simulink library "DiffSteer_model"  (R2013a)
settings: Solver=ode45  StartTime=0.0  StopTime=10.0  RelTol=1e-3
settings Model: Creator=Felipe  LastModifiedBy=Felipe

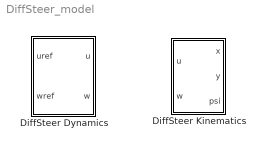
== system DiffSteer_model ==
  DiffSteer Dynamics : Subsystem  mask{umax=0.75, wmax=1.745, dumax=0.3, dwmax=1.745, param=[0.2604 0.2509 -0.000499 0.9965 0.00263 1.0768]}
      mask prompts: umax "Maximum linear velocity [m/s]"; wmax "Maximum angular velocity [rad/s]"; dumax "Maximum linear acceleration [m/s^2]"; dwmax "Maximum angular acceleration [rad/s^2]"; param "Dynamic parameters"
      mask help: Dynamics of the differential steered (unicycle-like) vehicle
      mask Help:
      | Dynamics of the differential steered (unicycle-like) vehicle.
      | 
      | This block recieves the linear and angular velocities signals (references) calculated by the robot controller and simulates the actual linear and angular velocities that the robot would have according to its dynamic parameters. It is intended to be used with the DiffSteer Kinematics block.
      | 
      | <b>Parameters:</b>
      | 
      | Maximum linear velocity (1x1): Vehicle linear velocity limit [m/s] (umax)
      | Maximum angular velocity (1x1): Vehicle angular velocity limit [rad/s] (wmax)
      | Maximum linear acceleration (1x1): Vehicle linear acceleration limit [m/s^2] (dumax)
      | Maximum angular acceleration (1x1): Vehicle angular acceleration limit [rad/s^2] (dwmax)
      | Dynamic parameters for an specific mobile robot acoording to [1-3] (1x6): (param)
      | [\theta_1 [s], \theta_2 [s], \theta_3 [sm/rad2], \theta_4, \theta_5 [s/m], \theta_6]
      | 
      | <b>Inputs::</b>
      | 
      | uref (1x1): reference for linear velocity [m/s]
      | wref (1x1): reference for angular velocity [rad/s]
      | 
      | <b>Outputs:</b>
      | 
      | u (1x1): robot linear velocity [m/s]
      | w (1x1): robot angular velocity [rad/s]
      | 
      | 
      | <b>Use:</b>
      | 
      | The inputs [uref, wref] must recieve the reference signals for linear and angular velocities.
      | 
      | The outputs [u, w] are to be conected to the inputs [u, w] of the Kinematics block.
      | 
      | 
      | <b>Notes:</b>
      | 
      | The default dynamic parameters correspond to the dynamics of the Pioneer 3-DX, from Mobile Robots, with a SICK LASER sensor mounted on its platform. To simulate the dynamics of a different robot, its parameters must be identified and input on the correspondent box.
      | 
      | The following sets of parameters were obtained via identification for some mobile robots:
      | 
      | [0.2604 0.2509 -0.000499 0.9965 0.00263 1.0768]; % Pioneer 3DX with Sick LASER sensor
      | [0.5338 0.2168 -0.0134 0.9560 -0.0843 1.0590]; % Pioneer 3DX without LASER sensor
      | [0.2183 0.1918 -0.0050 0.9993 -0.0279 1.0142]; % Pioneer 3DX (identified by Jeffrey Laut)
      | [0.1992 0.13736 0.001954 0.9907 0.01554 0.9866]; % Pioneer 2 without onboard computer (no LASER sensor)
      | [0.3037 0.2768 -0.0004018 0.9835 0.003818 1.0725]; % Pioneer 2 with onboard computer (no LASER sensor)
      | [0.3759 0.0188 0.0128 1.0027 -0.0015 0.9808]; % Robotic wheelchair carring a 55kg person
      | [0.4263 0.0289 0.0058 0.9883 0.0134 0.9931]; % Robotic wheelchair carring a 125kg person
      | [0.0228 0.0568 -0.0001 1.0030 0.0732 0.9981]; % Khepera III (identified by Jeffrey Laut)
      | 
      | For detailed information on the dynamic model and its parameters, please refer to:
      | 
      | [1] MARTINS, F.N., CARELLI, R., SARCINELLI-FILHO, M. and BASTOS-FILHO, T.F. Dynamic Modeling and Adaptive Dynamic Compensation for Unicycle-Like Mobile Robots. 14th International Conference on Advanced Robotics - ICAR 2009, Germany, June, 22-26, 2009.
      | 
      | [2] MARTINS, F.N., CELESTE, W.C., CARELLI, R., SARCINELLI-FILHO, M. and BASTOS-FILHO, T.F. An Adaptive Dynamic Controller for Autonomous Mobile Robot Trajectory Tracking. Control Engineering Practice, v. 16, p. 1354–1363, 2008. doi: 10.1016/j.conengprac.2008.03.004
      | 
      | [3] De La CRUZ, C., CARELLI, R. Dynamic model based formation control and obstacle avoidance of multi-robot systems. Robotica, n. 3, v. 26, p. 345--356, 2008.
      | 
      | [4] LAUT, Jeffrey. A Dynamic Parameter Identification Method for Migrating Control Strategies Between Heterogeneous Wheeled Mobile Robots. M.Sc. Diss. Worcester Polytechnic Institute, 2011.
  DiffSteer Kinematics : Subsystem  mask{x0=[0, 0, 0], a=0.2, umax=0.75, wmax=1.745, dumax=0.3, dwmax=1.745}
      mask prompts: x0 "Initial pose [x, y, psi]"; a "Distance from traction wheels axis center to the point of interest [m]"; umax "Maximum linear velocity [m/s]"; wmax "Maximum angular velocity [rad/s]"; dumax "Maximum linear acceleration [m/s^2]"; dwmax "Maximum angular acceleration [rad/s^2]"
      mask help: Kinematics of the differential steered vehicle
      mask Help:
      | Kinematics of the differential steered vehicle (unicycle-like).
      | 
      | A differential steered (or differential wheeled) robot has two separately driven wheels placed on either side of its structure. Its orientation is changed by varying the relative velocities of its wheels.
      | In this model, robot position [x,y] is the position of the point of interest, which is located on a distance "a" from the center of the line that connects both traction wheels. If a = 0, this model is equal to the unicycle.
      | 
      | <b>Parameters:</b>
      | 
      | Initial pose: Vehicle initial position and orientation on absolute reference frame [x_0, y_0, psi_0]
      | Distance between traction wheels axis and point of interest (1x1): a [m]
      | Maximum Linear velocity (1x1):  Vehicle speed limit [m/s] (umax)
      | Maximum Angular velocity (1x1):  Vehicle turning velocity limit [rad/s] (wmax)
      | Maximum linear acceleration (1x1): Vehicle linear acceleration limit [m/s2] (dumax)
      | Maximum angular acceleration (1x1): Vehicle angular acceleration limit [rad/s2] (dwmax)
      | 
      | 
      | <b>Inputs:</b>
      | 
      | u (1x1): reference for linear velocity [m/s]
      | w (1x1): reference for angular velocity [rad/s]
      | 
      | <b>Outputs:</b>
      | 
      | x (1x1): x-coordinate in world frame [m]
      | y (1x1): y-coordinate in world frame [m]
      | psi (1x1): heading angle in world frame [rad]
      | 
      | <b>Notes:</b>
      | 
      | 1. If a = 0, this model is equal to the unicycle.
      | 
      | 2. This model does not take into account the robot dynamics. It considers that the actual robot velocity is exactly equal to the reference velocity (if it is bellow its limit).
      | 
      | For more information on the robot kinematics and dynamics, please refer to:
      | 
      | [1] MARTINS, F.N., CARELLI, R., SARCINELLI-FILHO, M. and BASTOS-FILHO, T.F.
      | Dynamic Modeling and Adaptive Dynamic Compensation for Unicycle-Like
      | Mobile Robots. 14th International Conference on Advanced Robotics -
      | ICAR 2009, Germany, June, 22-26, 2009.
      | 
      | [2] MARTINS, F.N., CELESTE, W.C., CARELLI, R., SARCINELLI-FILHO, M. and
      | BASTOS-FILHO, T.F. An Adaptive Dynamic Controller for Autonomous Mobile Robot
      | Trajectory Tracking. Control Engineering Practice, v. 16, p. 1354–1363, 2008.
      | doi: 10.1016/j.conengprac.2008.03.004

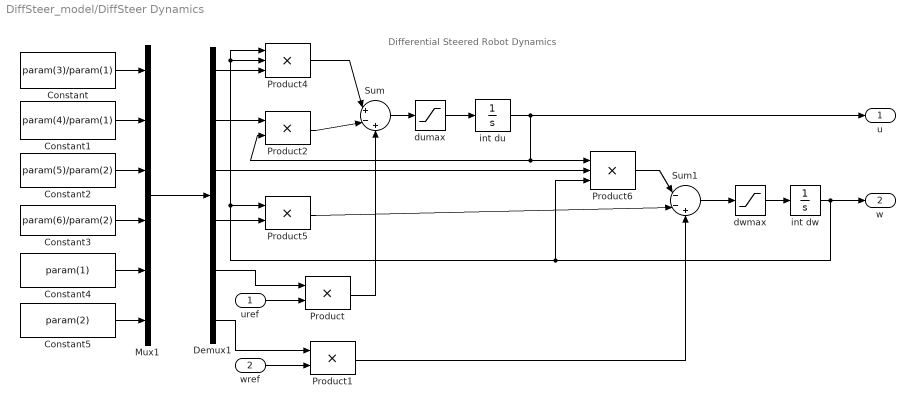
== system DiffSteer_model/DiffSteer Dynamics ==
  note: Differential Steered Robot Dynamics
  uref : Inport
  wref : Inport  Port=2
  Constant : Constant  Value=param(3)/param(1)
  Constant1 : Constant  Value=param(4)/param(1)
  Constant2 : Constant  Value=param(5)/param(2)
  Constant3 : Constant  Value=param(6)/param(2)
  Constant4 : Constant  Value=param(1)
  Constant5 : Constant  Value=param(2)
  Demux1 : Demux  Outputs=6
  Mux1 : Mux  Inputs=6
  Product{,1..2,5} (4 alike) : Product  SaturateOnIntegerOverflow=on  OutDataTypeStr=Inherit: Same as first input
  Product4 : Product  Inputs=3  SaturateOnIntegerOverflow=on  OutDataTypeStr=Inherit: Same as first input
  Product6 : Product  Inputs=3  SaturateOnIntegerOverflow=on  OutDataTypeStr=Inherit: Same as first input
  Sum : Sum  Inputs=|+-+  SaturateOnIntegerOverflow=on
  Sum1 : Sum  Inputs=|--+  SaturateOnIntegerOverflow=on
  dumax : Saturate  UpperLimit=dumax  LowerLimit=-dumax  ZeroCross=off
  dwmax : Saturate  UpperLimit=dwmax  LowerLimit=-dwmax  ZeroCross=off
  int du : Integrator  LimitOutput=on  UpperSaturationLimit=umax  LowerSaturationLimit=-umax
  int dw : Integrator  LimitOutput=on  UpperSaturationLimit=wmax  LowerSaturationLimit=-wmax
  u : Outport
  w : Outport  Port=2
  wires:
  Constant/1 -> Mux1/1
  Product1/1 -> Sum1/3
  Constant2/1 -> Mux1/3
  Demux1/4 -> Product5/2
  Demux1/5 -> Product/1
  Constant3/1 -> Mux1/4
  Constant1/1 -> Mux1/2
  Product4/1 -> Sum/1
  dwmax/1 -> int dw/1
  dumax/1 -> int du/1
  int du/1 -> u/1, Product2/2, Product6/1
  Demux1/6 -> Product1/1
  Constant5/1 -> Mux1/6
  Mux1/1 -> Demux1/1
  Constant4/1 -> Mux1/5
  Demux1/2 -> Product2/1
  Demux1/1 -> Product4/3
  Demux1/3 -> Product6/2
  int dw/1 -> w/1, Product6/3, Product5/1, Product4/1, Product4/2
  Product5/1 -> Sum1/2
  Product2/1 -> Sum/2
  Sum/1 -> dumax/1
  wref/1 -> Product1/2
  uref/1 -> Product/2
  Sum1/1 -> dwmax/1
  Product6/1 -> Sum1/1
  Product/1 -> Sum/3

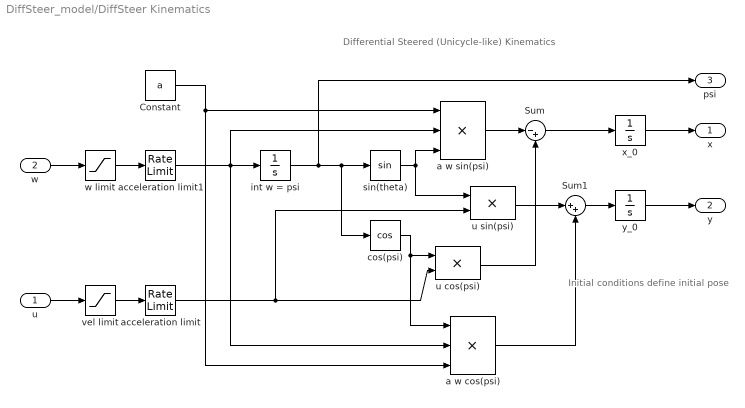
== system DiffSteer_model/DiffSteer Kinematics ==
  note: Initial conditions define
      | initial pose
  note: Differential Steered (Unicycle-like) Kinematics
  u : Inport
  w : Inport  Port=2
  Constant : Constant  Value=a
  Sum : Sum  Inputs=|-+  SaturateOnIntegerOverflow=on
  Sum1 : Sum  Inputs=|++  SaturateOnIntegerOverflow=on
  a w cos(psi) : Product  Inputs=3  SaturateOnIntegerOverflow=on  OutDataTypeStr=Inherit: Same as first input
  a w sin(psi) : Product  Inputs=3  SaturateOnIntegerOverflow=on  OutDataTypeStr=Inherit: Same as first input
  acceleration limit : RateLimiter  RisingSlewLimit=dumax  FallingSlewLimit=-dumax  SampleTimeMode=inherited
  acceleration limit1 : RateLimiter  RisingSlewLimit=dwmax  FallingSlewLimit=-dwmax  SampleTimeMode=inherited
  cos(psi) : Trigonometry  Operator=cos
  int w = psi : Integrator  InitialCondition=x0(3)
  sin(theta) : Trigonometry
  u cos(psi) : Product  SaturateOnIntegerOverflow=on  OutDataTypeStr=Inherit: Same as first input
  u sin(psi) : Product  SaturateOnIntegerOverflow=on  OutDataTypeStr=Inherit: Same as first input
  vel limit : Saturate  UpperLimit=umax  LowerLimit=-umax
  w limit : Saturate  UpperLimit=wmax  LowerLimit=-wmax
  x_0 : Integrator  InitialCondition=x0(1)
  y_0 : Integrator  InitialCondition=x0(2)
  x : Outport
  y : Outport  Port=2
  psi : Outport  Port=3
  wires:
  u sin(psi)/1 -> Sum1/1
  cos(psi)/1 -> u cos(psi)/1, a w cos(psi)/1
  acceleration limit1/1 -> a w cos(psi)/2, a w sin(psi)/2, int w = psi/1
  w limit/1 -> acceleration limit1/1
  Constant/1 -> a w sin(psi)/1, a w cos(psi)/3
  x_0/1 -> x/1
  u/1 -> vel limit/1
  Sum/1 -> x_0/1
  sin(theta)/1 -> a w sin(psi)/3, u sin(psi)/1
  a w cos(psi)/1 -> Sum1/2
  w/1 -> w limit/1
  int w = psi/1 -> psi/1, sin(theta)/1, cos(psi)/1
  vel limit/1 -> acceleration limit/1
  u cos(psi)/1 -> Sum/2
  acceleration limit/1 -> u sin(psi)/2, u cos(psi)/2
  a w sin(psi)/1 -> Sum/1
  Sum1/1 -> y_0/1
  y_0/1 -> y/1
